simulink subsystem "CorrectAngVelocity"  (R2021a)
settings: Solver=VariableStepAuto  StartTime=0.0  StopTime=10.0  RelTol=1e-3
settings Model: Creator=Laura  LastModifiedBy=Laura

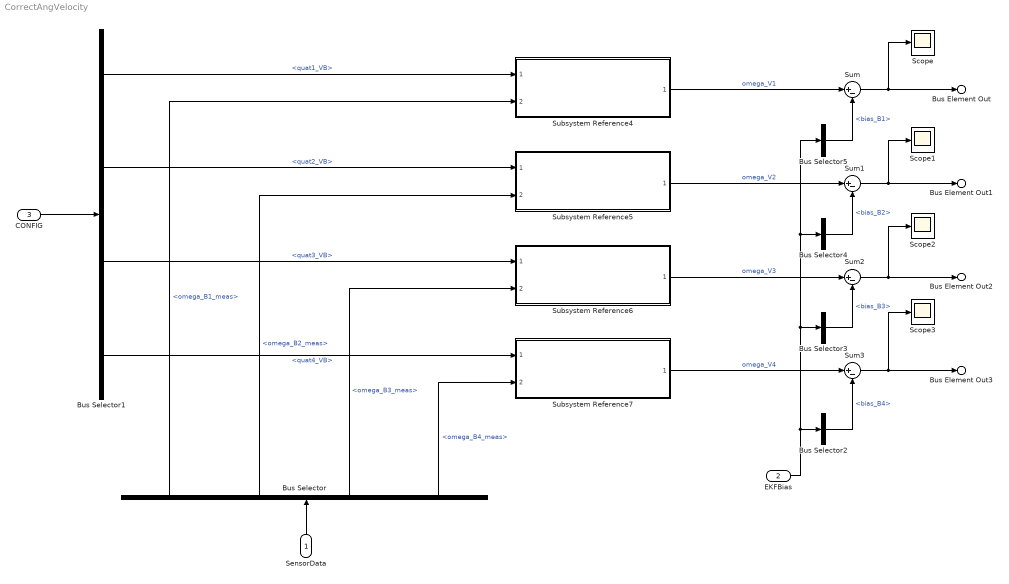
== system CorrectAngVelocity ==
  SensorData : Inport
  EKFBias : Inport  Port=2
  CONFIG : Inport  Port=3
  Bus Selector : BusSelector  OutputSignals=omega_B1_meas,omega_B2_meas,omega_B3_meas,omega_B4_meas
  Bus Selector1 : BusSelector  OutputSignals=quat1_VB,quat2_VB,quat3_VB,quat4_VB
  Bus Selector2 : BusSelector  OutputSignals=bias_B4
  Bus Selector3 : BusSelector  OutputSignals=bias_B3
  Bus Selector4 : BusSelector  OutputSignals=bias_B2
  Bus Selector5 : BusSelector  OutputSignals=bias_B1
  Scope{,1..3} (4 alike) : Scope
  Subsystem Reference{4..7} (4 alike) : Subsystem  ReferencedSubsystem=gyroSensor2CM
  Sum{,1..3} (4 alike) : Sum  Inputs=|+-
  Bus Element Out : Outport  PortName=EKFOmegaV_corrected  Element=omega_V1_corrected
  Bus Element Out1 : Outport  PortName=EKFOmegaV_corrected  Element=omega_V2_corrected
  Bus Element Out2 : Outport  PortName=EKFOmegaV_corrected  Element=omega_V3_corrected
  Bus Element Out3 : Outport  PortName=EKFOmegaV_corrected  Element=omega_V4_corrected
  wires:
  Subsystem Reference7/1 -> Sum3/1  "omega_V4"
  Subsystem Reference6/1 -> Sum2/1  "omega_V3"
  Subsystem Reference5/1 -> Sum1/1  "omega_V2"
  Subsystem Reference4/1 -> Sum/1  "omega_V1"
  Sum/1 -> Bus Element Out/1, Scope/1
  Bus Selector5/1 -> Sum/2  "<bias_B1>"
  Bus Selector4/1 -> Sum1/2  "<bias_B2>"
  Bus Selector3/1 -> Sum2/2  "<bias_B3>"
  Bus Selector2/1 -> Sum3/2  "<bias_B4>"
  EKFBias/1 -> Bus Selector3/1, Bus Selector5/1, Bus Selector4/1, Bus Selector2/1
  Bus Selector/1 -> Subsystem Reference4/2  "<omega_B1_meas>"
  Bus Selector/2 -> Subsystem Reference5/2  "<omega_B2_meas>"
  Bus Selector/3 -> Subsystem Reference6/2  "<omega_B3_meas>"
  Bus Selector/4 -> Subsystem Reference7/2  "<omega_B4_meas>"
  Bus Selector1/4 -> Subsystem Reference7/1  "<quat4_VB>"
  Bus Selector1/3 -> Subsystem Reference6/1  "<quat3_VB>"
  Bus Selector1/2 -> Subsystem Reference5/1  "<quat2_VB>"
  Bus Selector1/1 -> Subsystem Reference4/1  "<quat1_VB>"
  CONFIG/1 -> Bus Selector1/1
  SensorData/1 -> Bus Selector/1
  Sum1/1 -> Bus Element Out1/1, Scope1/1
  Sum2/1 -> Bus Element Out2/1, Scope2/1
  Sum3/1 -> Bus Element Out3/1, Scope3/1
